simulink model "reducedorderobserver"  (R2020a)
settings: Solver=VariableStepAuto  StartTime=0.0  StopTime=4  RelTol=1e-3
values from neighbouring files (symbols this model uses):
  A = [-6.30908 0 -10.9544 0 83.74458 0 0 24.05866 ... (first row only)    [project2.m]
  Aq = C1*A*L1 - K1*C*A*L1    [project2.m]
  B = BT'    [project2.m]
  Bq = C1*B - K1*C*B    [project2.m]
  c = rank(C)    [project2.m]
  C = [0 0 0 5.066579 -116.446 0 0 0 ... (first row only)    [project2.m]
  D = zeros(c, m)    [project2.m]
  F = place(A, B, dpoles)    [project2.m]
  K1 = K1T'    [project2.m]
  Kq = C1*A*L1*K1 + C1*A*L - K1*C*A*L - K1*C*A*L1*K1    [project2.m]
  L = Laug(1:n,1:c)    [project2.m]
  L1 = Laug(1:n,c+1:n)    [project2.m]
  m = rank(B)    [project2.m]
  r = n - c    [project2.m]
  x0 = [1 2 3 4 5 6 7 8]'    [project2.m]
  x0hat_reduced = eye(5)*L1'*(pinv(C'*C)*C'-(L+L1*K1))*y0    [project2.m]
settings Model: Creator=Alan  LastModifiedBy=Alan

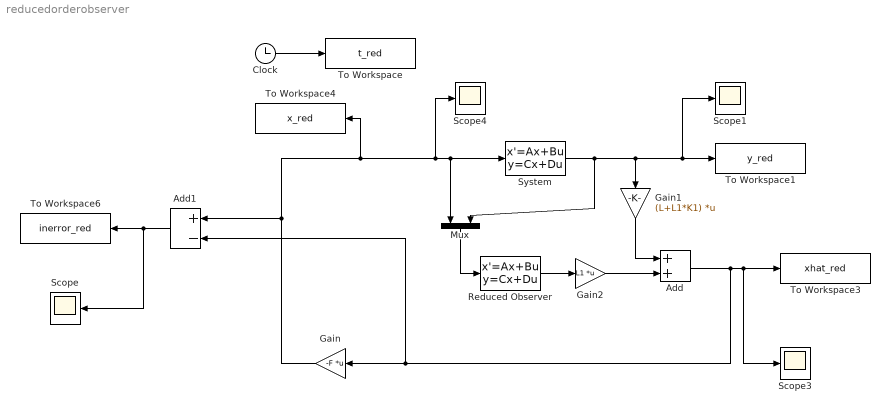
== system reducedorderobserver ==
  Add : Sum
  Add1 : Sum  Inputs=+-
  Clock : Clock
  Gain : Gain  Gain=-F  Multiplication=Matrix(K*u)
  Gain1 : Gain  Gain=(L+L1*K1)  Multiplication=Matrix(K*u)
  Gain2 : Gain  Gain=L1  Multiplication=Matrix(K*u)
  Mux : Mux  Inputs=2
  Reduced Observer : StateSpace  A=Aq  B=[Bq Kq]  C=eye(r)  D=zeros(r,m+c)  InitialCondition=x0hat_reduced
  Scope{,1,3..4} (4 alike) : Scope
  System : StateSpace  A=A  B=B  C=C  D=D  InitialCondition=x0
  To Workspace : ToWorkspace  VariableName=t_red  SaveFormat=Timeseries  SampleTime=-1
  To Workspace1 : ToWorkspace  VariableName=y_red  SaveFormat=Timeseries  SampleTime=-1
  To Workspace3 : ToWorkspace  VariableName=xhat_red  SaveFormat=Timeseries  SampleTime=-1
  To Workspace4 : ToWorkspace  VariableName=x_red  SaveFormat=Timeseries  SampleTime=-1
  To Workspace6 : ToWorkspace  VariableName=inerror_red  SaveFormat=Timeseries  SampleTime=-1
  wires:
  Add1/1 -> Scope/1, To Workspace6/1
  Gain/1 -> To Workspace4/1, Scope4/1, System/1, Mux/1, Add1/1
  System/1 -> Mux/2, Gain1/1, Scope1/1, To Workspace1/1
  Clock/1 -> To Workspace/1
  Gain2/1 -> Add/2
  Reduced Observer/1 -> Gain2/1
  Mux/1 -> Reduced Observer/1
  Gain1/1 -> Add/1
  Add/1 -> Add1/2, Gain/1, Scope3/1, To Workspace3/1
